simulink model "Task2_MaximumPowerTransfer"  (R2025b)
settings: Solver=VariableStepAuto  StartTime=0.0  StopTime=10  RelTol=1e-3
libraries: nesl_utility x6, fl_lib x5, simulink x1, ee_lib x1
settings Model: Creator=gdudgeon  LastModifiedBy=leona
settings RTWCC: GPUComputeCapability=3.5

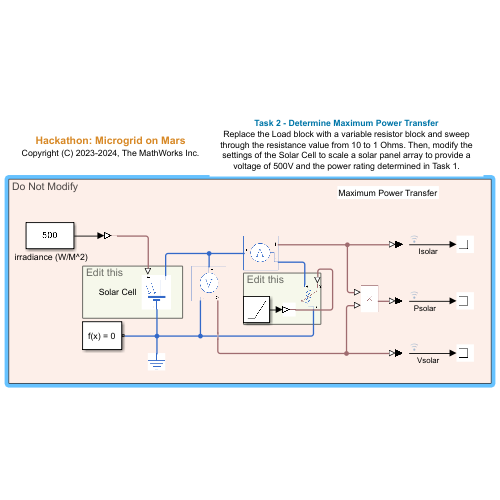
[thumbnail: Simulink's stored preview of the top-level diagram]
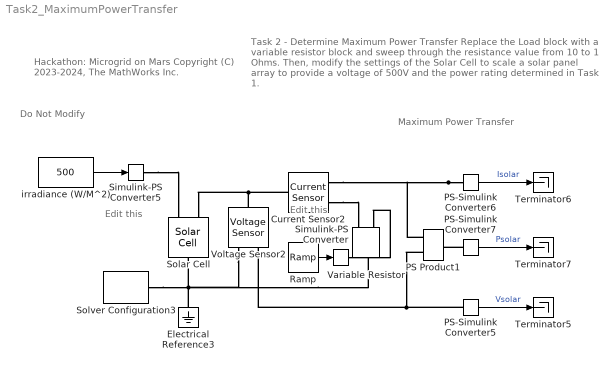
== system Task2_MaximumPowerTransfer ==
  note: Edit this
  note: Task 2 - Determine Maximum Power Transfer
      | Replace the Load block with a variable resistor block and sweep through the resistance value from 10 to 1 Ohms. Then, modify the settings of the Solar Cell to scale a solar panel array to provide a voltage of 500V and the power rating determined in Task 1.
  note: Hackathon: Microgrid on Mars
      | Copyright (C) 2023-2024, The MathWorks Inc.
  note: Maximum Power Transfer
  note: Do Not Modify
  note: Edit this
  " irradiance (W/M^2)" : Constant  Value=500
  Current Sensor2 : fl_lib/Electrical/Electrical Sensors/Current Sensor
  Electrical Reference3 : fl_lib/Electrical/Electrical Elements/Electrical Reference
  PS Product1 : fl_lib/Physical Signals/Functions/PS Product
  PS-Simulink Converter5 : nesl_utility/PS-Simulink Converter  PhysicalDomain=network_engine_domain  SubClassName=ps_output  LeftPortType=input  RightPortType=output  PseudoPeriodic=off  Frequencies=[]  VectorFormat=inherit  Unit=inherit  AffineConversion=off
  PS-Simulink Converter6 : nesl_utility/PS-Simulink Converter  PhysicalDomain=network_engine_domain  SubClassName=ps_output  LeftPortType=input  RightPortType=output  PseudoPeriodic=off  Frequencies=[]  VectorFormat=inherit  Unit=inherit  AffineConversion=off
  PS-Simulink Converter7 : nesl_utility/PS-Simulink Converter  PhysicalDomain=network_engine_domain  SubClassName=ps_output  LeftPortType=input  RightPortType=output  PseudoPeriodic=off  Frequencies=[]  VectorFormat=inherit  Unit=inherit  AffineConversion=off
  Ramp : simulink/Sources/Ramp  slope=1  start=0  InitialOutput=0
  Simulink-PS Converter : nesl_utility/Simulink-PS Converter  PhysicalDomain=network_engine_domain  SubClassName=ps_input  LeftPortType=input  RightPortType=output  PseudoPeriodic=off  Frequencies=[]  NoiseDistribution=none  NoiseParameters=[]  Unit=1  AffineConversion=off  FilteringAndDerivatives=provide  SimscapeFilterOrder=1  InputFilterTimeConstant=0.001  UdotUserProvided=0
  Simulink-PS Converter5 : nesl_utility/Simulink-PS Converter  PhysicalDomain=network_engine_domain  SubClassName=ps_input  LeftPortType=input  RightPortType=output  PseudoPeriodic=off  Frequencies=[]  NoiseDistribution=none  NoiseParameters=[]  Unit=W/m^2  AffineConversion=off  FilteringAndDerivatives=provide  SimscapeFilterOrder=1  InputFilterTimeConstant=0.001  UdotUserProvided=0
  Solar Cell : ee_lib/Sources/Solar Cell  prm=ee.enum.sources.solar_cell_prm.datasheet  Isc=10.6 A  Voc=0.61 V  Is=1e-6 A  Is2=0 A  Iph=7.34 A  Ir0=500 W/m^2  ec=1.5  N2=2  Rs=0 Ohm  Rp=inf Ohm  N_series=1000  N_parallel=10  TIPH1=0 1/K  EG=1.11 eV  TXIS1=3  TXIS2=3  TRS1=0  TRP1=0  Tmeas=25 degC  TFIXED=25 degC  thermal_mass=100 J/K  initial_temperature=25 degC
  Solver Configuration3 : nesl_utility/Solver Configuration  PhysicalDomain=network_engine_domain  SubClassName=solver  LeftPortType=input  RightPortType=generic  Tones=[]  Harmonics=[]  SimulateNoise=off  Profile=off  UseLocalSampling=off  EnableSwitchedLinearOptims=on  FrequencyDomain=off  UseCCode=off  RelTol=0.001  AbsTol=0.001  MinStep=1e-09  ToWorkspace=off  RevertToSquareIcSolve=off  NumHomotopyIterations=100  PhasorMode=off  PhasorModeNumHarmonics=1  ConsistencySolver=NEWTON_XTOL_AFTER_FTOL  IndexReductionMethod=None  DoDC=off  ResidualTolerance=1e-09  ConsistencyTolSource=GLOBAL  ConsistencyAbsTol=0.001  ConsistencyRelTol=0.001  ConsistencyTolFactor=0.001  UseLocalSolver=on  LocalSolverChoice=NE_BACKWARD_EULER_ADVANCER  ResolveIndetEquations=off  FunctionEvalNumThread=1  LocalSolverSampleTime=Ts  DoFixedCost=on  MaxNonlinIter=1  MaxModeIter=2  ComputeImpulses=off  ImpulseIterations=2  LinearAlgebra=Sparse  LinearAlgebraNumThread=0  EquationFormulation=NE_TIME_EF  DelaysMemoryBudget=1024  AutomaticFiltering=off  FilteringTimeConstant=0.001  PartitionStorageMethod=AS_NEEDED  PartitionMemoryBudget=1024  PartitionMethod=ROBUST  MultibodyUseLocalSolver=off  MultibodyLocalSolverChoice=ODE1  MultibodyLocalSolverSampleTime=0.001
  Terminator5 : Terminator
  Terminator6 : Terminator
  Terminator7 : Terminator
  Variable Resistor : fl_lib/Electrical/Electrical Elements/Variable Resistor  Rmin=5.07 Ohm  thermalEnable=false  thermal_mass=1 J/K  i_specify=off  i_priority=None  i=0 A  i_nominal_specify=off  i_nominal_value=1  i_nominal_unit=A  v_specify=off  v_priority=None  v=0 V  v_nominal_specify=off  v_nominal_value=1  v_nominal_unit=V  T_specify=off  T_priority=None  T=300 K  T_nominal_specify=off  T_nominal_value=1  T_nominal_unit=K
  Voltage Sensor2 : fl_lib/Electrical/Electrical Sensors/Voltage Sensor
  wires:
  PS-Simulink Converter5/1 -> Terminator5/1  "Vsolar"
  " irradiance (W/M^2)"/1 -> Simulink-PS Converter5/1
  PS-Simulink Converter6/1 -> Terminator6/1  "Isolar"
  PS-Simulink Converter7/1 -> Terminator7/1  "Psolar"
  Ramp/1 -> Simulink-PS Converter/1
  connections:
  Electrical Reference3/LConn1 -- Voltage Sensor2/RConn2 -- Variable Resistor/RConn1 -- Solver Configuration3/RConn1 -- Solar Cell/RConn1
  PS Product1/LConn2 -- PS-Simulink Converter5/LConn1 -- Voltage Sensor2/RConn1
  Current Sensor2/LConn1 -- Voltage Sensor2/LConn1 -- Solar Cell/LConn2
  PS-Simulink Converter6/LConn1 -- Current Sensor2/RConn1 -- PS Product1/LConn1
  Simulink-PS Converter5/RConn1 -- Solar Cell/LConn1
  Current Sensor2/RConn2 -- Variable Resistor/LConn2
  PS-Simulink Converter7/LConn1 -- PS Product1/RConn1
  Simulink-PS Converter/RConn1 -- Variable Resistor/LConn1
